simulink model "HW2_PR4"  (R2019a)
settings: Solver=ode23s  StartTime=0.0  StopTime=5  RelTol=1e-3
undefined symbols (not defined in the file or in its folder): g, I1, I2, l1, lc1, lc2, m1, m2
settings Model: Creator=canba  LastModifiedBy=canba

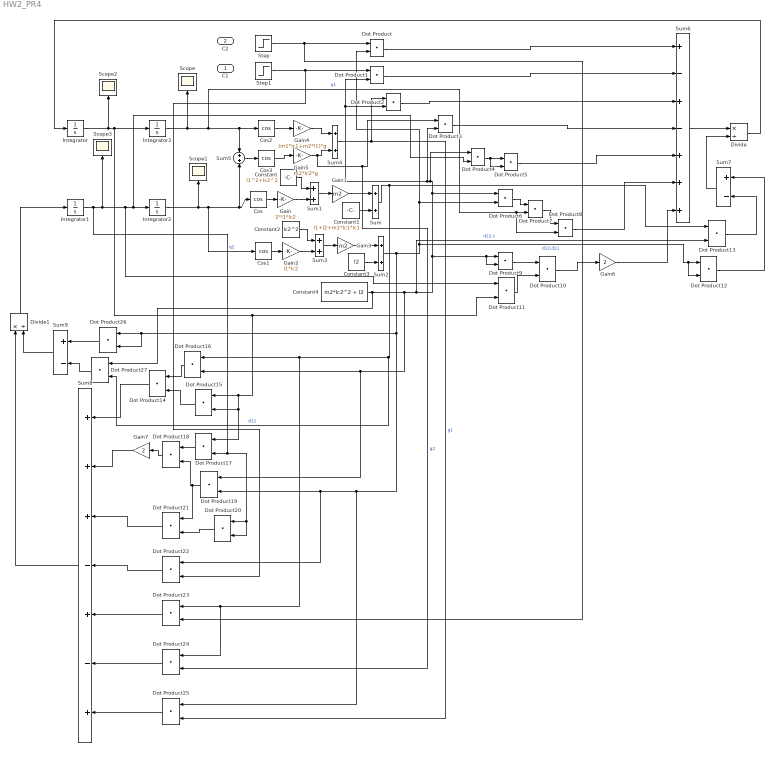
== system HW2_PR4 ==
  C1 : Inport
  C2 : Inport  Port=2
  Constant : Constant  Value=l1^2+lc2^2
  Constant1 : Constant  Value=I1+I2+m1*lc1*lc1
  Constant2 : Constant  Value=lc2^2
  Constant3 : Constant  Value=I2
  Constant4 : Constant  Value=m2*lc2^2 + I2
  Cos{,1..3} (4 alike) : Trigonometry  Operator=cos
  Divide : Product  Inputs=*/
  Divide1 : Product  Inputs=*/
  Dot Product{,1..27} (28 alike) : DotProduct  InputSameDT=on  OutDataTypeStr=Inherit: Inherit via internal rule
  Gain : Gain  Gain=2*l1*lc2
  Gain1 : Gain  Gain=m2
  Gain2 : Gain  Gain=l1*lc2
  Gain3 : Gain  Gain=m2
  Gain4 : Gain  Gain=(m1*lc1+m2*l1)*g
  Gain5 : Gain  Gain=m2*lc2*g
  Gain6 : Gain  Gain=2
  Gain7 : Gain  Gain=2
  Integrator : Integrator
  Integrator1 : Integrator
  Integrator2 : Integrator  InitialCondition=pi/6
  Integrator3 : Integrator  InitialCondition=pi/6
  Scope{,1..3} (4 alike) : Scope
  Step : Step  Time=0  SampleTime=0
  Step1 : Step  Time=0.2  SampleTime=0
  Sum{,1..4} (5 alike) : Sum
  Sum5 : Sum  Inputs=+|+
  Sum6 : Sum  Inputs=+-+-+++
  Sum7 : Sum  Inputs=+-
  Sum8 : Sum  Inputs=+++-+-+
  Sum9 : Sum  Inputs=+-
  wires:
  Sum/1 -> Dot Product27/2, Dot Product24/1, Dot Product23/1, Dot Product16/1, Dot Product13/1  "d11"
  Integrator/1 -> Scope2/1, Dot Product17/1, Dot Product15/2, Dot Product15/1, Dot Product11/2, Integrator3/1
  Integrator3/1 -> Scope/1, Dot Product8/2, Dot Product7/2, Sum5/1, Cos2/1  "q1"
  Cos/1 -> Gain/1
  Gain/1 -> Sum1/2
  Constant/1 -> Sum1/1
  Sum1/1 -> Gain1/1
  Gain1/1 -> Sum/1
  Constant1/1 -> Sum/2
  Constant3/1 -> Sum2/2
  Gain3/1 -> Sum2/1
  Sum3/1 -> Gain3/1
  Constant2/1 -> Sum3/1
  Gain2/1 -> Sum3/2
  Cos1/1 -> Gain2/1
  Integrator2/1 -> Scope1/1, Cos1/1, Sum5/2, Cos/1  "q2"
  Sum2/1 -> Dot Product6/2, Dot Product/2, Dot Product12/2, Dot Product12/1, Dot Product26/2, Dot Product26/1, Dot Product25/1, Dot Product22/1, Dot Product19/2  "d12,d21"
  Constant4/1 -> Dot Product27/1, Dot Product19/1, Dot Product16/2, Dot Product13/2, Dot Product6/1, Dot Product4/1, Dot Product3/2, Dot Product2/2, Dot Product1/2, Dot Product9/2, Dot Product9/1  "d22,c"
  Cos2/1 -> Gain4/1
  Sum5/1 -> Cos3/1
  Cos3/1 -> Gain5/1
  Gain4/1 -> Sum4/1
  Sum4/1 -> Dot Product25/2, Dot Product2/1  "g1"
  Gain5/1 -> Dot Product24/2, Dot Product3/1, Sum4/2  "g2"
  Step/1 -> Dot Product23/2, Dot Product/1
  Step1/1 -> Dot Product22/2, Dot Product1/1
  Dot Product1/1 -> Sum6/2
  Dot Product2/1 -> Sum6/3
  Dot Product3/1 -> Sum6/4
  Dot Product4/1 -> Dot Product5/2, Dot Product5/1
  Dot Product5/1 -> Sum6/5
  Dot Product6/1 -> Dot Product7/1
  Dot Product7/1 -> Dot Product8/1
  Dot Product8/1 -> Sum6/6
  Gain6/1 -> Sum6/7
  Dot Product9/1 -> Dot Product10/1
  Dot Product11/1 -> Dot Product10/2
  Dot Product10/1 -> Gain6/1
  Sum6/1 -> Divide/1
  Sum7/1 -> Divide/2
  Dot Product12/1 -> Sum7/1
  Dot Product13/1 -> Sum7/2
  Divide/1 -> Integrator/1
  Dot Product15/1 -> Dot Product14/2
  Dot Product16/1 -> Dot Product14/1
  Dot Product14/1 -> Sum8/1
  Dot Product17/1 -> Dot Product18/1
  Dot Product19/1 -> Dot Product21/1, Dot Product18/2
  Dot Product18/1 -> Gain7/1
  Gain7/1 -> Sum8/2
  Dot Product20/1 -> Dot Product21/2
  Dot Product21/1 -> Sum8/3
  Dot Product22/1 -> Sum8/4
  Dot Product23/1 -> Sum8/5
  Dot Product/1 -> Sum6/1
  Dot Product24/1 -> Sum8/6
  Dot Product25/1 -> Sum8/7
  Sum8/1 -> Divide1/1
  Divide1/1 -> Integrator1/1
  Dot Product26/1 -> Sum9/1
  Dot Product27/1 -> Sum9/2
  Sum9/1 -> Divide1/2
  Integrator1/1 -> Dot Product20/2, Dot Product20/1, Dot Product17/2, Dot Product11/1, Dot Product4/2, Integrator2/1, Scope3/1
